simulink model "Scalar"  (R2016a)
settings: Solver=FixedStepAuto  StartTime=0.0  StopTime=2  FixedStep=0.001  RelTol=1e-3
libraries: simulink x2
settings Model: Creator=gadis  LastModifiedBy=gadis

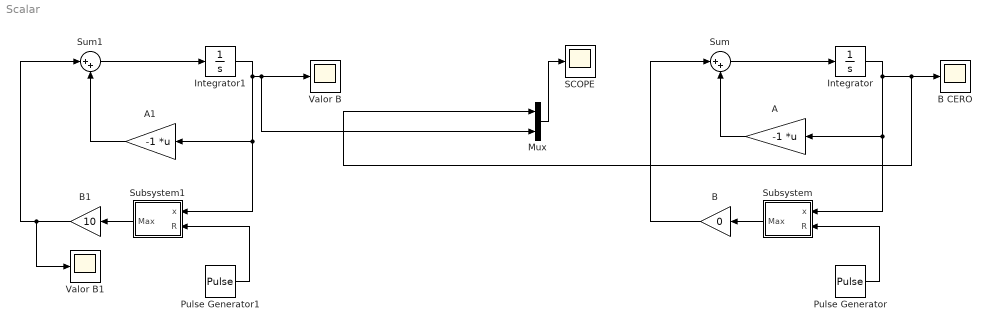
== system Scalar ==
  A : Gain  Gain=-1  Multiplication=Matrix(K*u) (u vector)
  A1 : Gain  Gain=-1  Multiplication=Matrix(K*u) (u vector)
  B : Gain  Gain=0
  B CERO : Scope
  B1 : Gain  Gain=10
  Integrator : Integrator  InitialCondition=1
  Integrator1 : Integrator  InitialCondition=-1
  Mux : Mux  Inputs=2
  Pulse Generator : DiscretePulseGenerator  PulseType=Time based  Period=0.1
  Pulse Generator1 : DiscretePulseGenerator  PulseType=Time based  Period=10  PulseWidth=10
  SCOPE : Scope
  Subsystem : Subsystem
  Subsystem1 : Subsystem
  Sum : Sum  Inputs=|++
  Sum1 : Sum  Inputs=|++
  Valor B : Scope
  Valor B1 : Scope
  wires:
  Sum/1 -> Integrator/1
  Integrator/1 -> Mux/1, B CERO/1, Subsystem/1(x), A/1
  A/1 -> Sum/2
  Subsystem/1(Max) -> B/1
  B/1 -> Sum/1
  Pulse Generator/1 -> Subsystem/2(R)
  Sum1/1 -> Integrator1/1
  Integrator1/1 -> A1/1, Subsystem1/1(x), Mux/2, Valor B/1
  A1/1 -> Sum1/2
  Subsystem1/1(Max) -> B1/1
  B1/1 -> Valor B1/1, Sum1/1
  Pulse Generator1/1 -> Subsystem1/2(R)
  Mux/1 -> SCOPE/1

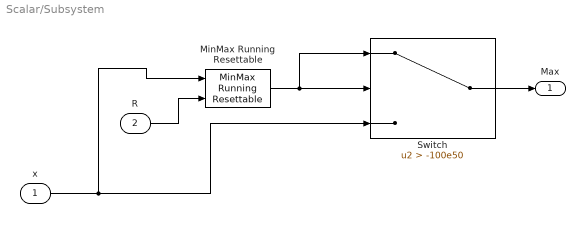
== system Scalar/Subsystem ==
  x : Inport
  R : Inport  Port=2
  MinMax Running Resettable : simulink/Math Operations/MinMax Running Resettable  Function=max  vinit=-inf
  Switch : Switch  Criteria=u2 > Threshold  Threshold=-100e50
  Max : Outport
  wires:
  MinMax Running Resettable/1 -> Switch/1, Switch/2
  Switch/1 -> Max/1
  R/1 -> MinMax Running Resettable/2
  x/1 -> Switch/3, MinMax Running Resettable/1

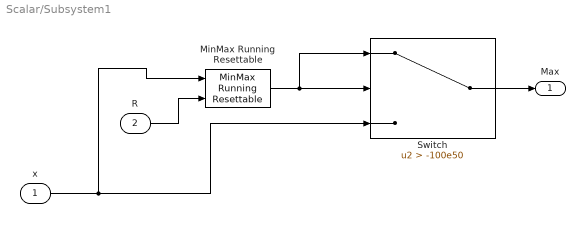
== system Scalar/Subsystem1 ==
  x : Inport
  R : Inport  Port=2
  MinMax Running Resettable : simulink/Math Operations/MinMax Running Resettable  Function=max  vinit=-inf
  Switch : Switch  Criteria=u2 > Threshold  Threshold=-100e50
  Max : Outport
  wires:
  x/1 -> MinMax Running Resettable/1, Switch/3
  R/1 -> MinMax Running Resettable/2
  Switch/1 -> Max/1
  MinMax Running Resettable/1 -> Switch/2, Switch/1
